simulink model "staticDecouplingControl"  (R2017b)
settings: Solver=VariableStepAuto  StartTime=0.0  StopTime=time  RelTol=1e-3
values from neighbouring files (symbols this model uses):
  d = 0.15    [runStatic.m]
  Kp = eye(2)    [runDynamic.m]    (also in runStatic.m)
  L = 0.13    [runDynamic.m]    (also in runLyapunov.m; runStatic.m)
  L_controller = 0.13    [runDynamic.m]    (also in runLyapunov.m = 0.143; runStatic.m)
  R = 2    [runDynamic.m]    (also in runLyapunov.m; runStatic.m)
  r = 0.1    [runDynamic.m]    (also in runLyapunov.m; runStatic.m)
  r_controller = 0.1    [runDynamic.m]    (also in runLyapunov.m; runStatic.m)
  satMax = inf    [runDynamic.m]    (also in runLyapunov.m; runStatic.m)
  satMin = -inf    [runDynamic.m]    (also in runLyapunov.m; runStatic.m)
  wd = 0.5    [runDynamic.m]    (also in runLyapunov.m; runStatic.m)
  Xi = [2.3; 0; pi]    [runDynamic.m]    (also in runLyapunov.m; runStatic.m)
settings Model: Creator=yleni  LastModifiedBy=yleni

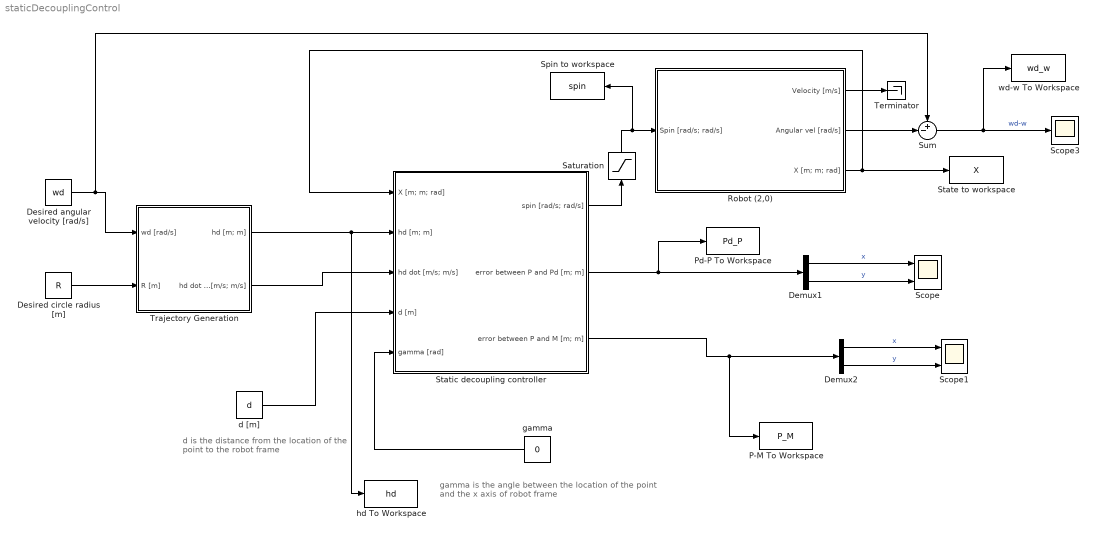
== system staticDecouplingControl ==
  note: gamma is the angle between the location
      | of the point and the x axis of robot frame
  note: d is the distance from the location
      | of the point to the robot frame
  Demux1 : Demux  Outputs=2
  Demux2 : Demux  Outputs=2
  Desired angular velocity [rad/s] : Constant  Value=wd
  Desired circle radius [m] : Constant  Value=R
  P-M To Workspace : ToWorkspace  VariableName=P_M  SampleTime=-1
      settings: Save2DSignal=2-D array (concatenate along first dimension)
  Pd-P To Workspace : ToWorkspace  VariableName=Pd_P  SampleTime=-1
      settings: Save2DSignal=2-D array (concatenate along first dimension)
  Robot (2,0) : Subsystem  mask{r=r, L=L, Xstart=Xi}
      mask prompts: r "Wheel radius [m]"; L "Distance from the wheel to the robot frame center [m]"; Xstart "Initial conditions [m; m; rad]"
  Saturation : Saturate  UpperLimit=satMax  LowerLimit=satMin
  Scope : Scope  NumInputPorts=2
  Scope1 : Scope  NumInputPorts=2
  Scope3 : Scope
  Spin to workspace : ToWorkspace  VariableName=spin  SampleTime=-1
      settings: Save2DSignal=2-D array (concatenate along first dimension)
  State to workspace : ToWorkspace  VariableName=X  SampleTime=-1
      settings: Save2DSignal=2-D array (concatenate along first dimension)
  Static decoupling controller : Subsystem  mask{Kp=Kp, L=L_controller, r=r_controller}
      mask prompts: Kp "Gain position control law"; L "Distance from the wheel to the robot frame center [m]"; r "Wheel radius [m]"
  Sum : Sum  Inputs=+-|
  Terminator : Terminator
  Trajectory Generation : Subsystem
  d [m] : Constant  Value=d
  gamma : Constant  Value=0
  hd To Workspace : ToWorkspace  VariableName=hd  SampleTime=-1
      settings: Save2DSignal=2-D array (concatenate along first dimension)
  wd-w To Workspace : ToWorkspace  VariableName=wd_w  SampleTime=-1
      settings: Save2DSignal=2-D array (concatenate along first dimension)
  wires:
  Static decoupling controller/1(spin [rad/s; rad/s]) -> Saturation/1
  Trajectory Generation/2(hd dot [m/s; m/s]) -> Static decoupling controller/3(hd dot [m/s; m/s])
  Robot (2,0)/3(X [m; m; rad]) -> State to workspace/1, Static decoupling controller/1(X [m; m; rad])
  d [m]/1 -> Static decoupling controller/4(d [m])
  gamma/1 -> Static decoupling controller/5(gamma [rad])
  Desired angular velocity [rad/s]/1 -> Sum/1, Trajectory Generation/1(wd [rad/s])
  Desired circle radius [m]/1 -> Trajectory Generation/2(R [m])
  Demux1/1 -> Scope/1  "x"
  Demux1/2 -> Scope/2  "y"
  Demux2/2 -> Scope1/2  "y"
  Static decoupling controller/3(error between P and M [m; m]) -> P-M To Workspace/1, Demux2/1
  Demux2/1 -> Scope1/1  "x"
  Robot (2,0)/2(Angular vel [rad/s]) -> Sum/2
  Sum/1 -> wd-w To Workspace/1, Scope3/1  "wd-w"
  Trajectory Generation/1(hd [m; m]) -> hd To Workspace/1, Static decoupling controller/2(hd [m; m])
  Saturation/1 -> Spin to workspace/1, Robot (2,0)/1(Spin [rad/s; rad/s])
  Static decoupling controller/2("error between P and Pd [m; m] ") -> Pd-P To Workspace/1, Demux1/1
  Robot (2,0)/1(Velocity [m/s]) -> Terminator/1

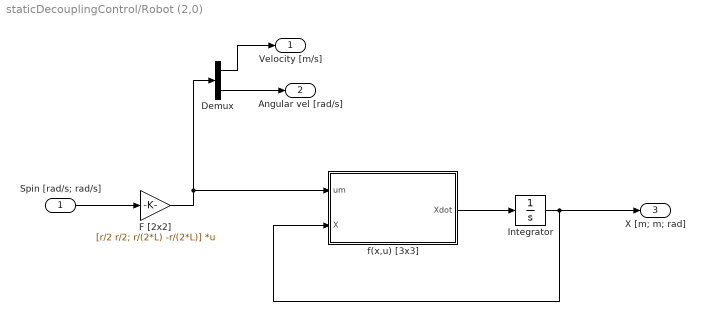
== system staticDecouplingControl/Robot (2,0) ==
  Spin [rad/s; rad/s] : Inport
  Demux : Demux  Outputs=2
  F [2x2] : Gain  Gain=[r/2 r/2; r/(2*L) -r/(2*L)]  Multiplication=Matrix(K*u)
  Integrator : Integrator  InitialCondition=Xstart
  f(x,u) [3x3] : MATLAB Function  TreatAsAtomicUnit=on
  Velocity [m/s] : Outport
  Angular vel [rad/s] : Outport  Port=2
  X [m; m; rad] : Outport  Port=3
  wires:
  f(x,u) [3x3]/1(Xdot) -> Integrator/1
  F [2x2]/1 -> f(x,u) [3x3]/1(um), Demux/1
  Demux/2 -> Angular vel [rad/s]/1
  Demux/1 -> Velocity [m/s]/1
  Integrator/1 -> X [m; m; rad]/1, f(x,u) [3x3]/2(X)
  Spin [rad/s; rad/s]/1 -> F [2x2]/1

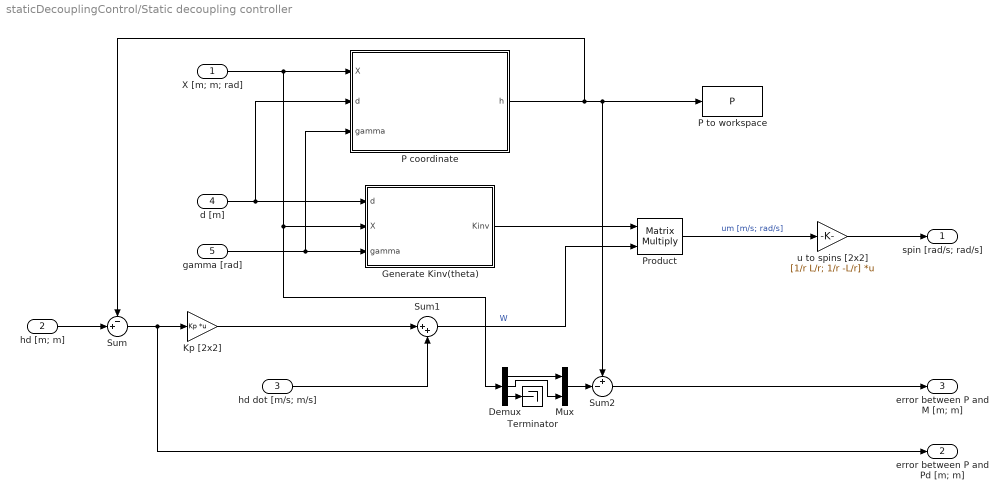
== system staticDecouplingControl/Static decoupling controller ==
  X [m; m; rad] : Inport
  hd [m; m] : Inport  Port=2
  hd dot [m/s; m/s] : Inport  Port=3
  d [m] : Inport  Port=4
  gamma [rad] : Inport  Port=5
  Demux : Demux  Outputs=3
  Generate Kinv(theta) : MATLAB Function  TreatAsAtomicUnit=on
  Kp [2x2] : Gain  Gain=Kp  Multiplication=Matrix(K*u)
  Mux : Mux  Inputs=2
  P coordinate : MATLAB Function  TreatAsAtomicUnit=on
  P to workspace : ToWorkspace  VariableName=P  SampleTime=-1
      settings: Save2DSignal=2-D array (concatenate along first dimension)
  Product : Product  Multiplication=Matrix(*)
  Sum : Sum  Inputs=-+|
  Sum1 : Sum  Inputs=|++
  Sum2 : Sum  Inputs=+-|
  Terminator : Terminator
  u to spins [2x2] : Gain  Gain=[1/r L/r; 1/r -L/r]  Multiplication=Matrix(K*u)
  spin [rad/s; rad/s] : Outport
  "error between P and Pd [m; m] " : Outport  Port=2
  error between P and M [m; m] : Outport  Port=3
  wires:
  X [m; m; rad]/1 -> Demux/1, Generate Kinv(theta)/2(X), P coordinate/1(X)
  Generate Kinv(theta)/1(Kinv) -> Product/1
  P coordinate/1(h) -> P to workspace/1, Sum2/1, Sum/1
  Sum/1 -> "error between P and Pd [m; m] "/1, Kp [2x2]/1
  Kp [2x2]/1 -> Sum1/1
  Product/1 -> u to spins [2x2]/1  "um [m/s; rad/s]"
  Sum1/1 -> Product/2  "W"
  hd [m; m]/1 -> Sum/2
  hd dot [m/s; m/s]/1 -> Sum1/2
  d [m]/1 -> P coordinate/2(d), Generate Kinv(theta)/1(d)
  gamma [rad]/1 -> P coordinate/3(gamma), Generate Kinv(theta)/3(gamma)
  u to spins [2x2]/1 -> spin [rad/s; rad/s]/1
  Demux/1 -> Mux/1
  Demux/2 -> Mux/2
  Mux/1 -> Sum2/2
  Sum2/1 -> error between P and M [m; m]/1
  Demux/3 -> Terminator/1

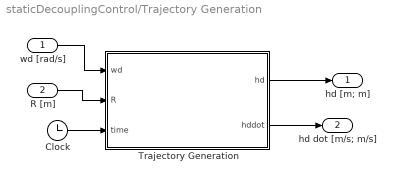
== system staticDecouplingControl/Trajectory Generation ==
  wd [rad/s] : Inport
  R [m] : Inport  Port=2
  Clock : Clock
  Trajectory Generation : MATLAB Function  TreatAsAtomicUnit=on
  hd [m; m] : Outport
  hd dot [m/s; m/s] : Outport  Port=2
  wires:
  wd [rad/s]/1 -> Trajectory Generation/1(wd)
  Trajectory Generation/2(hddot) -> hd dot [m/s; m/s]/1
  R [m]/1 -> Trajectory Generation/2(R)
  Trajectory Generation/1(hd) -> hd [m; m]/1
  Clock/1 -> Trajectory Generation/3(time)

== matlab function staticDecouplingControl/Static decoupling controller/Generate Kinv(theta) ==
  data: d input; X input; Kinv output; gamma input
function Kinv = generateKinv(d, X, gamma)

K = [cos(X(3)) -d*sin(X(3)+gamma); sin(X(3)) d*cos(X(3)+gamma)];
Kinv = inv(K);

== matlab function staticDecouplingControl/Robot (2,0)/f(x,u) [3x3] ==
  data: um input; Xdot output; X input
function Xdot  = evolutionModel(um, X)

Xdot = zeros(3,1);
Xdot(1) = um(1) * cos(X(3));
Xdot(2) = um(1) * sin(X(3));
Xdot(3) = um(2);

== matlab function staticDecouplingControl/Trajectory Generation/Trajectory Generation ==
  data: wd input; hd output; R input; time input; hddot output
function [hd, hddot] = trajectoryGeneration(wd, R, time)

hd = [R*cos(wd*time); R*sin(wd*time)];

hddot = [-R*sin(wd*time)*wd; R*cos(wd*time)*wd];

== matlab function staticDecouplingControl/Static decoupling controller/P coordinate ==
  data: X input; h output; d input; gamma input
function h = coordinateP(X ,d, gamma)

h = [X(1)+d*cos(X(3)+gamma); X(2)+d*sin(X(3)+gamma)];
